simulink model "s2dot3_43lookup"  (R2023b)
settings: Solver=VariableStepAuto  StartTime=0.0  StopTime=20  RelTol=1e-3
settings Model: Creator=lxj  LastModifiedBy=lxj

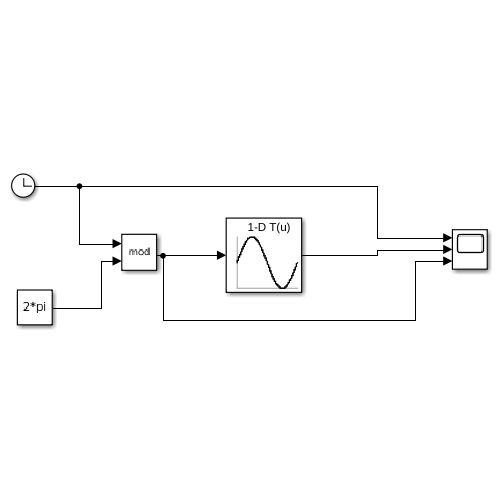
[thumbnail: Simulink's stored preview of the top-level diagram]
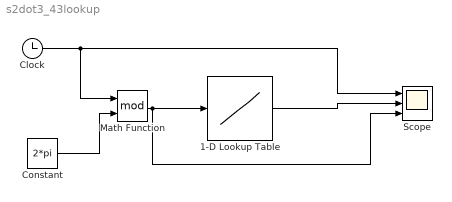
== system s2dot3_43lookup ==
  1-D Lookup Table : Lookup_n-D  NumberOfTableDimensions=1  BreakpointsForDimension1=linspace(0,2*pi,256)  Table=sin(linspace(0,2*pi,256))  InternalRulePriority=Speed  RndMeth=Simplest
  Clock : Clock
  Constant : Constant  Value=2*pi
  Math Function : Math  Operator=mod
  Scope : Scope  NumInputPorts=3
  wires:
  Clock/1 -> Scope/1, Math Function/1
  Constant/1 -> Math Function/2
  1-D Lookup Table/1 -> Scope/2
  Math Function/1 -> Scope/3, 1-D Lookup Table/1
